simulink library "Kitchen_Lib"  (R2023a)
settings: Solver=VariableStepAuto  StartTime=0.0  StopTime=10.0  RelTol=1e-3  EnableMultiTasking=on
undefined symbols (not defined in the file): Kitc_BusTyp_P, Kitc_BusTypSkyr_C, Kitc_ColrLedColrls_C, Kitc_ColrLedGrn_C, Kitc_ColrLedRed_C, Kitc_ColrLedYlw_C, Kitc_StDgnWtrTank_C, Kitc_StElecPlugScktOffByClmp50_P, Kitc_StsDlyBlink_C, Kitc_StsErrBlink_C, Kitc_StsFctAcvn_P, Kitc_StsInfoBlink_C, Kitc_StsKitchnOffAutoIgOff_P, Kitc_StsKitchnOffBySwt_P, Kitc_StsKitchnOffDoorLockd_P, Kitc_StsKitchnOffIgOff_P, Kitc_StsKitchnOffUv_P, Kitc_StsKitchnOnBySwt_P, Kitc_StsKitchnOnNVM_P, Kitc_StsLedOff_C, Kitc_StsLedOn_C, Kitc_StsLrgCnsAcv_P, Kitc_StTrfrAnSwtInstd_P, Kitc_StTrfrSwtInstd_P, Kitc_TiKitcRefgtrOffDly_P, Kitc_ULowrThdBat_C, Kitc_UUpprThdBat_C, Kitc_ValFalse_C, Kitc_ValPwmFreq2_C, Kitc_ValPwmFreq_C, Kitc_ValTrue_C
libraries: MAN_Library x50, E2E_Lib x3
(part 6 of 13)

== system Kitchen_Lib/Kitchen/100ms/Kitchn/Subsystem1/Subsystem19/KitchenEnable/KitchenOnBySwitch ==
  Kitc_StKitcSwtUpprPart : Inport
  "GW_ModeExbn " : Inport  Port=2
  "GW_StUvTopPrio " : Inport  Port=3
  Kitchn_On : Inport  Port=4
  Logical Operator : Logic  Inputs=4  AllPortsSameDT=off  OutDataTypeStr=boolean
  Logical Operator1 : Logic  Operator=NOT  Inputs=4  AllPortsSameDT=off  OutDataTypeStr=boolean
  Logical Operator2 : Logic  Operator=NOT  Inputs=4  AllPortsSameDT=off  OutDataTypeStr=boolean
  Logical Operator3 : Logic  Operator=NOT  Inputs=4  AllPortsSameDT=off  OutDataTypeStr=boolean
  "KitchnOnBySwt " : Outport
  tag scope: Kitc_StKitcSwtUpprPart=global
  wires:
  Kitc_StKitcSwtUpprPart/1 -> [Kitc_StKitcSwtUpprPart], Logical Operator/1
  "GW_StUvTopPrio "/1 -> Logical Operator2/1
  Logical Operator/1 -> "KitchnOnBySwt "/1
  "GW_ModeExbn "/1 -> Logical Operator1/1
  Logical Operator2/1 -> Logical Operator/3
  Logical Operator3/1 -> Logical Operator/4
  Logical Operator1/1 -> Logical Operator/2
  Kitchn_On/1 -> Logical Operator3/1

== system Kitchen_Lib/Kitchen/100ms/Kitchn/Subsystem1/Subsystem19/KitchenEnable/KitchenOnNVM ==
  "GW_StStrtNew " : Inport
  "GW_ModeExbn " : Inport  Port=2
  GW_StClmp15 : Inport  Port=3
  Kitchen_On : Inport  Port=4
  KitchnOffBySwt : Inport  Port=5
  HostsSideBotmBtn_OFF : Inport  Port=6
  Kitc_ModeKitcNv : DataStoreWrite  DataStoreName=Kitc_ModeKitcNv  IndexOptions=Index vector (dialog)  Indices=1  OutputSizes=1
  Kitc_ModeKitcNv1 : DataStoreRead  DataStoreName=Kitc_ModeKitcNv  IndexOptions=Index vector (dialog)  Indices=1  OutputSizes=1
  Logical Operator32 : Logic  Inputs=5  AllPortsSameDT=off  OutDataTypeStr=boolean
  Logical Operator33 : Logic  Operator=NOT  Inputs=4  AllPortsSameDT=off  OutDataTypeStr=boolean
  Logical Operator34 : Logic  Operator=NOT  Inputs=4  AllPortsSameDT=off  OutDataTypeStr=boolean
  Logical Operator35 : Logic  Operator=NOT  Inputs=4  AllPortsSameDT=off  OutDataTypeStr=boolean
  NVM : Subsystem
  NvM_ActiveOnlyForFirstCycle : Subsystem  AncestorBlock=MAN_Library/NvM_ActiveOnlyForFirstCycle
  RisingEdgeDetection5 : Subsystem  AncestorBlock=MAN_Library/RisingEdgeDetection
  "KitchnOnNVM  " : Outport
  wires:
  "GW_ModeExbn "/1 -> Logical Operator34/1
  Logical Operator33/1 -> Logical Operator32/2
  RisingEdgeDetection5/1(Q) -> Logical Operator32/1
  Logical Operator35/1 -> Logical Operator32/5
  "GW_StStrtNew "/1 -> NVM/3("GW_StStrtNew "), Logical Operator35/1
  Logical Operator34/1 -> Logical Operator32/3
  Logical Operator32/1 -> Kitc_ModeKitcNv/1, "KitchnOnNVM  "/1
  Kitchen_On/1 -> Logical Operator33/1, NVM/5(Kitchn_On)
  Kitc_ModeKitcNv1/1 -> NvM_ActiveOnlyForFirstCycle/1(NVM_Bool_In)
  GW_StClmp15/1 -> RisingEdgeDetection5/1(CLK), NVM/6(GW_StClmp15)
  KitchnOffBySwt/1 -> NVM/1(KitchnOffBySwt)
  HostsSideBotmBtn_OFF/1 -> NVM/2(HostsSideBotmBtn_OFF)
  NvM_ActiveOnlyForFirstCycle/1(NVM_Bool_Out) -> NVM/4(Kitc_ModeKitcNv), Logical Operator32/4

== system Kitchen_Lib/Kitchen/100ms/Kitchn/Subsystem1/Subsystem19/KitchenEnable/Subsystem ==
  StateChange : Inport
  Ground : Ground
  Logical Operator : Logic  AllPortsSameDT=off  OutDataTypeStr=boolean
  RS : Subsystem  AncestorBlock=MAN_Library/RS
  RisingEdgeDetection : Subsystem  AncestorBlock=MAN_Library/RisingEdgeDetection
  StateChangePulse : Subsystem  AncestorBlock=MAN_Library/StateChangePulse
  Terminator : Terminator
  Terminator1 : Terminator
  TimeConstant : Subsystem  AncestorBlock=MAN_Library/TimeConstant  mask{hours=0, minutes=0, seconds=0, miliseconds=0}
      mask prompts: hours "Hour"
      mask DialogControl TimeConstant Prompt: Time Constant
      mask Display:
      | timeDraw = 'Time#';
      | if( hours == 0 && minutes == 0 && seconds == 0 && miliseconds == 0)
      |     timeDraw = strcat(timeDraw,'0secs'),
      | else
      |     if( hours ~= 0)
      |         timeDraw = strcat(timeDraw,num2str(hours),'hours');
      |     end
      |     if( minutes ~= 0)
      |         timeDraw = strcat(timeDraw,num2str(minutes),'min');
      |     end
      |     if( seconds ~= 0)
      |         timeDraw = strcat(timeDraw,num2str(seconds),'sec');
      |     end
      |     if( miliseconds ~= 0)
      |         timeDraw = strcat(timeDraw,num2str(miliseconds),'ms');
      |     end
      | end
      | fprintf(timeDraw);
  TurnOnDelay : Subsystem  AncestorBlock=MAN_Library/TurnOnDelay  mask(Turn On Delay){CycleTime=Cycle Time: 10 Ms}
      mask prompts: CycleTime "Select the Cycle Time:"
      mask help:
      | This is an EDGE DELAY where the turning-on edge is delayed. The delay period is entered at input PT. Output Q is set on TRUE after turning on input IN, only after the delay period is over. Output ET counts the time - beginning with the occurrence of the positive edge - until the value set at PT has been reached. The output ET shows the expired time since turning input IN on until the input state of IN is put through to output Q.
      |
      | IN : Timer starting bit
      | PT : Preset time of timer
      | Q  : Time up flag
      | ET : Current value of timer
      mask TypeOptions CycleTime: Cycle Time: 1 Ms | Cycle Time: 10 Ms | Cycle Time: 100 Ms | Cycle Time: 1000 Ms
      mask Display:
      | disp('{\bf\fontsize{18}Turn On Delay}', 'texmode','on');
      | 
      | port_label('input', 1,'IN');
      | port_label('input', 2,'PT');
      | port_label('output',1,'Q');
      | port_label('output',2,'ET');
  Unit Delay : UnitDelay  SampleTime=-1  HasFrameUpgradeWarning=on
  Kitchn_On : Outport
  wires:
  RS/1(Q) -> TurnOnDelay/1(TurnOnDelayEnable), Kitchn_On/1
  TimeConstant/1(time) -> TurnOnDelay/2(TurnOnDelayThreshold)
  TurnOnDelay/2(TurnOnDelayExpiredTime) -> Terminator/1
  TurnOnDelay/1(TurnOnDelayFlag) -> Unit Delay/1
  Unit Delay/1 -> Logical Operator/2
  Logical Operator/1 -> RS/2(R)
  RisingEdgeDetection/1(Q) -> Logical Operator/1, RS/1(S)
  StateChange/1 -> RisingEdgeDetection/1(CLK)
  Ground/1 -> StateChangePulse/1(IN)
  StateChangePulse/1(OUT) -> Terminator1/1

== system Kitchen_Lib/Kitchen/100ms/Kitchn/Subsystem1/Subsystem19/KitchenSwtLed/HostessError ==
  HostSideButtonLock : Inport
  Kitc_WarnLrgCns : Inport  Port=2
  Kitc_BusTypSkyr : Inport  Port=3
  Logical Operator14 : Logic  AllPortsSameDT=off  OutDataTypeStr=boolean
  Logical Operator15 : Logic  Operator=NOT  Inputs=4  AllPortsSameDT=off  OutDataTypeStr=boolean
  Multiport Switch3 : MultiPortSwitch  DataPortOrder=Zero-based contiguous  Inputs=2  zeroidx=on  SaturateOnIntegerOverflow=off  InputSameDT=off
  HosstesErr : Outport
  wires:
  Kitc_BusTypSkyr/1 -> Multiport Switch3/1
  HostSideButtonLock/1 -> Multiport Switch3/3, Logical Operator14/2
  Multiport Switch3/1 -> HosstesErr/1
  Logical Operator14/1 -> Multiport Switch3/2
  Logical Operator15/1 -> Logical Operator14/1
  Kitc_WarnLrgCns/1 -> Logical Operator15/1

== system Kitchen_Lib/Kitchen/100ms/Kitchn/Subsystem1/Subsystem19/KitchenSwtLed/HostessGreenDelay ==
  LrgCns : Inport
  Kitchn_On : Inport  Port=2
  Kitc_WarnLrgCns : Inport  Port=3
  HostSideButtonLock : Inport  Port=4
  HostsCallAcv : Inport  Port=5
  Kitc_BusTypSkyr : Inport  Port=6
  Constant2 : Constant  Value=Kitc_ValFalse_C
  Data Type Conversion : DataTypeConversion  OutDataTypeStr=uint8  SaturateOnIntegerOverflow=off  RndMeth=Floor
  Logical Operator{8..11} (4 alike) : Logic  Operator=NOT  Inputs=4  AllPortsSameDT=off  OutDataTypeStr=boolean
  Logical Operator7 : Logic  Inputs=5  AllPortsSameDT=off  OutDataTypeStr=boolean
  Multiport Switch4 : MultiPortSwitch  DataPortOrder=Zero-based contiguous  Inputs=2  zeroidx=on  SaturateOnIntegerOverflow=off  InputSameDT=off
  HostessGreenDly : Outport
  wires:
  Kitc_BusTypSkyr/1 -> Multiport Switch4/1
  Multiport Switch4/1 -> HostessGreenDly/1
  HostsCallAcv/1 -> Logical Operator10/1
  Kitchn_On/1 -> Logical Operator7/3
  Logical Operator8/1 -> Logical Operator7/5
  LrgCns/1 -> Logical Operator9/1
  Logical Operator9/1 -> Logical Operator7/2
  Logical Operator10/1 -> Logical Operator7/4
  Logical Operator11/1 -> Logical Operator7/1
  Kitc_WarnLrgCns/1 -> Logical Operator11/1
  Constant2/1 -> Data Type Conversion/1
  Data Type Conversion/1 -> Multiport Switch4/3
  Logical Operator7/1 -> Multiport Switch4/2
  HostSideButtonLock/1 -> Logical Operator8/1

== system Kitchen_Lib/Kitchen/100ms/Kitchn/Subsystem1/Subsystem19/KitchenSwtLed/HostessGreenOn ==
  LrgCns : Inport
  Kitchn_On : Inport  Port=2
  Kitc_WarnLrgCns : Inport  Port=3
  HostSideButtonLock : Inport  Port=4
  HostsCallAcv : Inport  Port=5
  Kitc_BusTypSkyr : Inport  Port=6
  Logical Operator1 : Logic  Inputs=4  AllPortsSameDT=off  OutDataTypeStr=boolean
  Logical Operator{2..5,54} (5 alike) : Logic  Operator=NOT  Inputs=4  AllPortsSameDT=off  OutDataTypeStr=boolean
  Logical Operator52 : Logic  Inputs=3  AllPortsSameDT=off  OutDataTypeStr=boolean
  Multiport Switch4 : MultiPortSwitch  DataPortOrder=Zero-based contiguous  Inputs=2  zeroidx=on  SaturateOnIntegerOverflow=off  InputSameDT=off
  HostessGreenOn : Outport
  wires:
  Kitc_BusTypSkyr/1 -> Multiport Switch4/1
  Multiport Switch4/1 -> HostessGreenOn/1
  HostsCallAcv/1 -> Logical Operator54/1, Logical Operator3/1
  Kitchn_On/1 -> Logical Operator52/1
  Logical Operator52/1 -> Multiport Switch4/3
  Logical Operator54/1 -> Logical Operator52/3
  HostSideButtonLock/1 -> Logical Operator5/1, Logical Operator4/1
  Logical Operator1/1 -> Multiport Switch4/2
  LrgCns/1 -> Logical Operator1/1
  Logical Operator2/1 -> Logical Operator1/2
  Logical Operator3/1 -> Logical Operator1/3
  Kitc_WarnLrgCns/1 -> Logical Operator2/1
  Logical Operator4/1 -> Logical Operator1/4
  Logical Operator5/1 -> Logical Operator52/2

== system Kitchen_Lib/Kitchen/100ms/Kitchn/Subsystem1/Subsystem19/KitchenSwtLed/HostessRed ==
  Kitc_WarnLrgCns : Inport
  HostSideButtonLock : Inport  Port=2
  HostsCallAcv : Inport  Port=3
  Kitc_BusTypSkyr : Inport  Port=4
  Logical Operator12 : Logic  AllPortsSameDT=off  OutDataTypeStr=boolean
  Logical Operator13 : Logic  Operator=NOT  Inputs=4  AllPortsSameDT=off  OutDataTypeStr=boolean
  Logical Operator5 : Logic  AllPortsSameDT=off  OutDataTypeStr=boolean
  Logical Operator8 : Logic  Operator=NOT  Inputs=4  AllPortsSameDT=off  OutDataTypeStr=boolean
  Multiport Switch4 : MultiPortSwitch  DataPortOrder=Zero-based contiguous  Inputs=2  zeroidx=on  SaturateOnIntegerOverflow=off  InputSameDT=off
  HostessRed : Outport
  wires:
  Kitc_BusTypSkyr/1 -> Multiport Switch4/1
  Multiport Switch4/1 -> HostessRed/1
  Logical Operator5/1 -> Multiport Switch4/3, Logical Operator12/2
  HostsCallAcv/1 -> Logical Operator5/1
  Logical Operator8/1 -> Logical Operator5/2
  Logical Operator12/1 -> Multiport Switch4/2
  Logical Operator13/1 -> Logical Operator12/1
  Kitc_WarnLrgCns/1 -> Logical Operator13/1
  HostSideButtonLock/1 -> Logical Operator8/1

== system Kitchen_Lib/Kitchen/100ms/Kitchn/Subsystem1/Subsystem19/KitchenSwtLed/KitchenError ==
  note: TFoE
  "GW_ModeExbn " : Inport
  "GW_StUvTopPrio " : Inport  Port=2
  In3 : Inport  Port=3
  Kitc_StKitcSwtUpprPart : Inport  Port=4
  Kitc_WarnLrgCns : Inport  Port=5
  Kitc_BusTypSkyr : Inport  Port=6
  Logical Operator21 : Logic  Operator=NOT  Inputs=4  AllPortsSameDT=off  OutDataTypeStr=boolean
  Logical Operator22 : Logic  AllPortsSameDT=off  OutDataTypeStr=boolean
  Logical Operator23 : Logic  Operator=NOT  Inputs=4  AllPortsSameDT=off  OutDataTypeStr=boolean
  Logical Operator4 : Logic  Inputs=3  AllPortsSameDT=off  OutDataTypeStr=boolean
  Multiport Switch6 : MultiPortSwitch  DataPortOrder=Zero-based contiguous  Inputs=2  zeroidx=on  SaturateOnIntegerOverflow=off  InputSameDT=off
  RisingEdgeDetection : Subsystem  AncestorBlock=MAN_Library/RisingEdgeDetection
  Terminator3 : Terminator
  TurnOffDelay : Subsystem  AncestorBlock=MAN_Library/TurnOffDelay  mask(Turn Off Delay){CycleTime=Cycle Time: 10 Ms}
      mask prompts: CycleTime "Select the Cycle Time:"
      mask help:
      | This is an EDGE DELAY where the turning-off edge is delayed. The delay period is entered at input PT. The output Q is reset after turning off input IN, only after the delay period is over. Output ET counts the time - beginning with the occurrence of the negative edge - until the value set at PT has been reached. The output ET shows the expired time since turning input IN off until the input state of IN is put through to output Q.
      |
      | IN : Timer starting bit
      | PT : Preset time of timer
      | Q  : Time pulse flag
      | ET : Current value of timer
      mask TypeOptions CycleTime: Cycle Time: 1 Ms | Cycle Time: 10 Ms | Cycle Time: 100 Ms | Cycle Time: 1000 Ms
      mask Display:
      | disp('{\bf\fontsize{18}Turn Off Delay}', 'texmode','on');
      | 
      | port_label('input', 1,'IN');
      | port_label('input', 2,'PT');
      | port_label('output',1,'Q');
      | port_label('output',2,'ET');
  KitchenErr : Outport
  wires:
  In3/1 -> TurnOffDelay/2(TurnOffDelayThreshold)
  TurnOffDelay/1(TurnOffDelayFlag) -> Logical Operator22/2, Multiport Switch6/3
  Kitc_StKitcSwtUpprPart/1 -> RisingEdgeDetection/1(CLK)
  "GW_StUvTopPrio "/1 -> Logical Operator4/2
  "GW_ModeExbn "/1 -> Logical Operator21/1
  Logical Operator4/1 -> TurnOffDelay/1(TurnOffDelayEnable)
  RisingEdgeDetection/1(Q) -> Logical Operator4/3
  Logical Operator21/1 -> Logical Operator4/1
  Multiport Switch6/1 -> KitchenErr/1
  Logical Operator23/1 -> Logical Operator22/1
  Logical Operator22/1 -> Multiport Switch6/2
  Kitc_WarnLrgCns/1 -> Logical Operator23/1
  Kitc_BusTypSkyr/1 -> Multiport Switch6/1
  TurnOffDelay/2(TurnOffDelayExpiredTime) -> Terminator3/1

== system Kitchen_Lib/Kitchen/100ms/Kitchn/Subsystem1/Subsystem19/KitchenSwtLed/KitchenGreenLed ==
  LrgCns : Inport
  Kitchn_On : Inport  Port=2
  Kitc_WarnLrgCns : Inport  Port=3
  Kitc_BusTypSkyr : Inport  Port=4
  Logical Operator16 : Logic  AllPortsSameDT=off  OutDataTypeStr=boolean
  Logical Operator17 : Logic  Operator=NOT  Inputs=4  AllPortsSameDT=off  OutDataTypeStr=boolean
  Multiport Switch4 : MultiPortSwitch  DataPortOrder=Zero-based contiguous  Inputs=2  zeroidx=on  SaturateOnIntegerOverflow=off  InputSameDT=off
  KitchenGreenOn : Outport
  wires:
  Kitchn_On/1 -> Multiport Switch4/3
  LrgCns/1 -> Logical Operator16/1
  Kitc_BusTypSkyr/1 -> Multiport Switch4/1
  Logical Operator16/1 -> Multiport Switch4/2
  Logical Operator17/1 -> Logical Operator16/2
  Kitc_WarnLrgCns/1 -> Logical Operator17/1
  Multiport Switch4/1 -> KitchenGreenOn/1

== system Kitchen_Lib/Kitchen/100ms/Kitchn/Subsystem1/Subsystem19/KitchenSwtLed/KitchenGreenLedDelay ==
  LrgCns : Inport
  Kitchn_On : Inport  Port=2
  Kitc_WarnLrgCns : Inport  Port=3
  Kitc_BusTypSkyr : Inport  Port=4
  Constant7 : Constant  Value=Kitc_ValFalse_C
  Data Type Conversion1 : DataTypeConversion  OutDataTypeStr=uint8  SaturateOnIntegerOverflow=off  RndMeth=Floor
  Logical Operator18 : Logic  Inputs=3  AllPortsSameDT=off  OutDataTypeStr=boolean
  Logical Operator19 : Logic  Operator=NOT  Inputs=4  AllPortsSameDT=off  OutDataTypeStr=boolean
  Logical Operator20 : Logic  Operator=NOT  Inputs=4  AllPortsSameDT=off  OutDataTypeStr=boolean
  Multiport Switch4 : MultiPortSwitch  DataPortOrder=Zero-based contiguous  Inputs=2  zeroidx=on  SaturateOnIntegerOverflow=off  InputSameDT=off
  KitchenGreenDly : Outport
  wires:
  Kitc_BusTypSkyr/1 -> Multiport Switch4/1
  Logical Operator18/1 -> Multiport Switch4/2
  Multiport Switch4/1 -> KitchenGreenDly/1
  Kitchn_On/1 -> Logical Operator18/1
  LrgCns/1 -> Logical Operator19/1
  Logical Operator19/1 -> Logical Operator18/3
  Logical Operator20/1 -> Logical Operator18/2
  Kitc_WarnLrgCns/1 -> Logical Operator20/1
  Constant7/1 -> Data Type Conversion1/1
  Data Type Conversion1/1 -> Multiport Switch4/3

== system Kitchen_Lib/Kitchen/100ms/Kitchn/Subsystem1/Subsystem19/KitchenSwtLed/KitchenYellowLed ==
  Kitc_WarnLrgCns : Inport
  Kitc_BusTypSkyr : Inport  Port=2
  Constant11 : Constant  Value=Kitc_ValFalse_C
  Data Type Conversion2 : DataTypeConversion  OutDataTypeStr=uint8  SaturateOnIntegerOverflow=off  RndMeth=Floor
  Multiport Switch7 : MultiPortSwitch  DataPortOrder=Zero-based contiguous  Inputs=2  zeroidx=on  SaturateOnIntegerOverflow=off  InputSameDT=off
  KitchenYellow : Outport
  wires:
  Kitc_BusTypSkyr/1 -> Multiport Switch7/1
  Data Type Conversion2/1 -> Multiport Switch7/3
  Multiport Switch7/1 -> KitchenYellow/1
  Kitc_WarnLrgCns/1 -> Multiport Switch7/2
  Constant11/1 -> Data Type Conversion2/1

== system Kitchen_Lib/Kitchen/100ms/Kitchn/Subsystem1/Subsystem19/KitchenSwtLed/LEDSignal_Subsytem ==
  note: Output Led SignalValue
      | Led Signal Blink Info
      | Led Signal Color Info
      |
      | 0
      | Off
      |
      | 1
      | 200/800
      |
      | green
      |
      | 2
      | 250/250
      |
      | green
      |
      | 3
      | 800/200
      |
      | green
      |
      | 4
      | 100%
      |
      | green
      |
      | 5
      | 200/800
      | yellow
      |
      | 6
      | 250/250
      | yellow
      |
      | 7
      | 800/200
      |
      | yellow
      |
      | 8
      | 100%
      |
      | yellow
      |
      | 9
      | 200/800
      | red
      |
      | 10
      | 250/250
      | red
      |
      | 11
      | 800/200
      |
      | red
      |
      | 12
      | 100%
      |
      | red
      |
      | 14
      | Error
      |
      | 15
      | NA
  note: Off
  note: Blink Info
      | Value
      |
      | Led off
      | 0
      |
      | Led on
      | 1
      |
      | Led 500ms on 500ms off
      | 2
      |
      | Led 250ms on 250ms off
      | 3
      |
      | Led200ms on 800ms off
      | 4
      |
      | Led 800ms on 200ms off
      | 5
  note: Led Info
      | Value
      |
      | Yellow
      | 2
      |
      | Green
      | 3
      |
      | Red
      | 1
  note: 800/200
  note: 500/500
  note: 200/800
  note: 250/250
  note: 100
  note: 800/200
  note: 500/500
  note: 200/800
  note: 250/250
  note: 100
  note: 800/200
  note: 500/500
  note: 200/800
  note: 250/250
  note: 100
  note: Off
  note: Off
  Color : Inport
  Status : Inport  Port=2
  Error : Inport  Port=3
  NA : Inport  Port=4
  Constant{1..5,56,61,66} (8 alike) : Constant  Value=uint8(0)
  Constant55 : Constant  Value=uint8(4)
  Constant57 : Constant  Value=uint8(2)
  Constant58 : Constant  Value=uint8(1)
  Constant59 : Constant  Value=uint8(3)
  Constant60 : Constant  Value=uint8(8)
  Constant62 : Constant  Value=uint8(6)
  Constant63 : Constant  Value=uint8(5)
  Constant64 : Constant  Value=uint8(7)
  Constant65 : Constant  Value=uint8(12)
  Constant67 : Constant  Value=uint8(10)
  Constant68 : Constant  Value=uint8(9)
  Constant69 : Constant  Value=uint8(11)
  Constant70 : Constant  Value=uint8(14)
  Constant71 : Constant  Value=uint8(16)
  Ground : Ground
  Ground1 : Ground
  Ground2 : Ground
  Multiport Switch17 : MultiPortSwitch  DataPortOrder=Zero-based contiguous  Inputs=6  DataPortForDefault=Additional data port  zeroidx=on  SaturateOnIntegerOverflow=off  InputSameDT=off
  Multiport Switch23 : MultiPortSwitch  DataPortOrder=Zero-based contiguous  Inputs=4  DataPortForDefault=Additional data port  DiagnosticForDefault=None  zeroidx=on  SaturateOnIntegerOverflow=off  InputSameDT=off
  Multiport Switch24 : MultiPortSwitch  DataPortOrder=Zero-based contiguous  Inputs=6  DataPortForDefault=Additional data port  zeroidx=on  SaturateOnIntegerOverflow=off  InputSameDT=off
  Multiport Switch25 : MultiPortSwitch  DataPortOrder=Zero-based contiguous  Inputs=6  DataPortForDefault=Additional data port  zeroidx=on  SaturateOnIntegerOverflow=off  InputSameDT=off
  Multiport Switch26 : MultiPortSwitch  DataPortOrder=Zero-based contiguous  Inputs=2  zeroidx=on  SaturateOnIntegerOverflow=off  InputSameDT=off
  Multiport Switch27 : MultiPortSwitch  DataPortOrder=Zero-based contiguous  Inputs=2  zeroidx=on  SaturateOnIntegerOverflow=off  InputSameDT=off
  Led : Outport
  wires:
  Status/1 -> Multiport Switch25/1, Multiport Switch24/1, Multiport Switch17/1
  Multiport Switch17/1 -> Multiport Switch23/5
  Multiport Switch24/1 -> Multiport Switch23/4
  Multiport Switch25/1 -> Multiport Switch23/3
  Constant1/1 -> Multiport Switch23/6
  Constant5/1 -> Multiport Switch23/2
  Constant57/1 -> Multiport Switch17/5
  Constant64/1 -> Multiport Switch24/7
  Ground1/1 -> Multiport Switch24/4
  Constant60/1 -> Multiport Switch24/3
  Constant62/1 -> Multiport Switch24/5
  Constant63/1 -> Multiport Switch24/6
  Constant61/1 -> Multiport Switch24/2
  Multiport Switch26/1 -> Multiport Switch27/2
  Multiport Switch23/1 -> Multiport Switch26/2
  Error/1 -> Multiport Switch26/1
  Constant69/1 -> Multiport Switch25/7
  Constant67/1 -> Multiport Switch25/5
  Ground2/1 -> Multiport Switch25/4
  Constant66/1 -> Multiport Switch25/2
  Constant68/1 -> Multiport Switch25/6
  Constant65/1 -> Multiport Switch25/3
  Constant70/1 -> Multiport Switch26/3
  Constant71/1 -> Multiport Switch27/3
  Color/1 -> Multiport Switch23/1
  Constant58/1 -> Multiport Switch17/6
  Constant55/1 -> Multiport Switch17/3
  NA/1 -> Multiport Switch27/1
  Constant56/1 -> Multiport Switch17/2
  Ground/1 -> Multiport Switch17/4
  Constant59/1 -> Multiport Switch17/7
  Multiport Switch27/1 -> Led/1
  Constant2/1 -> Multiport Switch24/8
  Constant3/1 -> Multiport Switch17/8
  Constant4/1 -> Multiport Switch25/8

== system Kitchen_Lib/Kitchen/100ms/Kitchn/Subsystem1/Subsystem19/KitchenSwtLed/LEDSignal_Subsytem1 ==
  note: Output Led SignalValue
      | Led Signal Blink Info
      | Led Signal Color Info
      |
      | 0
      | Off
      |
      | 1
      | 200/800
      |
      | green
      |
      | 2
      | 250/250
      |
      | green
      |
      | 3
      | 800/200
      |
      | green
      |
      | 4
      | 100%
      |
      | green
      |
      | 5
      | 200/800
      | yellow
      |
      | 6
      | 250/250
      | yellow
      |
      | 7
      | 800/200
      |
      | yellow
      |
      | 8
      | 100%
      |
      | yellow
      |
      | 9
      | 200/800
      | red
      |
      | 10
      | 250/250
      | red
      |
      | 11
      | 800/200
      |
      | red
      |
      | 12
      | 100%
      |
      | red
      |
      | 14
      | Error
      |
      | 15
      | NA
  note: Off
  note: Blink Info
      | Value
      |
      | Led off
      | 0
      |
      | Led on
      | 1
      |
      | Led 500ms on 500ms off
      | 2
      |
      | Led 250ms on 250ms off
      | 3
      |
      | Led200ms on 800ms off
      | 4
      |
      | Led 800ms on 200ms off
      | 5
  note: Led Info
      | Value
      |
      | Yellow
      | 2
      |
      | Green
      | 3
      |
      | Red
      | 1
  note: 800/200
  note: 500/500
  note: 200/800
  note: 250/250
  note: 100
  note: 800/200
  note: 500/500
  note: 200/800
  note: 250/250
  note: 100
  note: 800/200
  note: 500/500
  note: 200/800
  note: 250/250
  note: 100
  note: Off
  note: Off
  Color : Inport
  Status : Inport  Port=2
  Error : Inport  Port=3
  NA : Inport  Port=4
  Constant{1..5,56,61,66} (8 alike) : Constant  Value=uint8(0)
  Constant55 : Constant  Value=uint8(4)
  Constant57 : Constant  Value=uint8(2)
  Constant58 : Constant  Value=uint8(1)
  Constant59 : Constant  Value=uint8(3)
  Constant60 : Constant  Value=uint8(8)
  Constant62 : Constant  Value=uint8(6)
  Constant63 : Constant  Value=uint8(5)
  Constant64 : Constant  Value=uint8(7)
  Constant65 : Constant  Value=uint8(12)
  Constant67 : Constant  Value=uint8(10)
  Constant68 : Constant  Value=uint8(9)
  Constant69 : Constant  Value=uint8(11)
  Constant70 : Constant  Value=uint8(14)
  Constant71 : Constant  Value=uint8(16)
  Ground : Ground
  Ground1 : Ground
  Ground2 : Ground
  Multiport Switch17 : MultiPortSwitch  DataPortOrder=Zero-based contiguous  Inputs=6  DataPortForDefault=Additional data port  zeroidx=on  SaturateOnIntegerOverflow=off  InputSameDT=off
  Multiport Switch23 : MultiPortSwitch  DataPortOrder=Zero-based contiguous  Inputs=4  DataPortForDefault=Additional data port  DiagnosticForDefault=None  zeroidx=on  SaturateOnIntegerOverflow=off  InputSameDT=off
  Multiport Switch24 : MultiPortSwitch  DataPortOrder=Zero-based contiguous  Inputs=6  DataPortForDefault=Additional data port  zeroidx=on  SaturateOnIntegerOverflow=off  InputSameDT=off
  Multiport Switch25 : MultiPortSwitch  DataPortOrder=Zero-based contiguous  Inputs=6  DataPortForDefault=Additional data port  zeroidx=on  SaturateOnIntegerOverflow=off  InputSameDT=off
  Multiport Switch26 : MultiPortSwitch  DataPortOrder=Zero-based contiguous  Inputs=2  zeroidx=on  SaturateOnIntegerOverflow=off  InputSameDT=off
  Multiport Switch27 : MultiPortSwitch  DataPortOrder=Zero-based contiguous  Inputs=2  zeroidx=on  SaturateOnIntegerOverflow=off  InputSameDT=off
  Led : Outport
  wires:
  Status/1 -> Multiport Switch25/1, Multiport Switch24/1, Multiport Switch17/1
  Multiport Switch17/1 -> Multiport Switch23/5
  Multiport Switch24/1 -> Multiport Switch23/4
  Multiport Switch25/1 -> Multiport Switch23/3
  Constant1/1 -> Multiport Switch23/6
  Constant5/1 -> Multiport Switch23/2
  Constant57/1 -> Multiport Switch17/5
  Constant64/1 -> Multiport Switch24/7
  Ground1/1 -> Multiport Switch24/4
  Constant60/1 -> Multiport Switch24/3
  Constant62/1 -> Multiport Switch24/5
  Constant63/1 -> Multiport Switch24/6
  Constant61/1 -> Multiport Switch24/2
  Multiport Switch26/1 -> Multiport Switch27/2
  Multiport Switch23/1 -> Multiport Switch26/2
  Error/1 -> Multiport Switch26/1
  Constant69/1 -> Multiport Switch25/7
  Constant67/1 -> Multiport Switch25/5
  Ground2/1 -> Multiport Switch25/4
  Constant66/1 -> Multiport Switch25/2
  Constant68/1 -> Multiport Switch25/6
  Constant65/1 -> Multiport Switch25/3
  Constant70/1 -> Multiport Switch26/3
  Constant71/1 -> Multiport Switch27/3
  Color/1 -> Multiport Switch23/1
  Constant58/1 -> Multiport Switch17/6
  Constant55/1 -> Multiport Switch17/3
  NA/1 -> Multiport Switch27/1
  Constant56/1 -> Multiport Switch17/2
  Ground/1 -> Multiport Switch17/4
  Constant59/1 -> Multiport Switch17/7
  Multiport Switch27/1 -> Led/1
  Constant2/1 -> Multiport Switch24/8
  Constant3/1 -> Multiport Switch17/8
  Constant4/1 -> Multiport Switch25/8

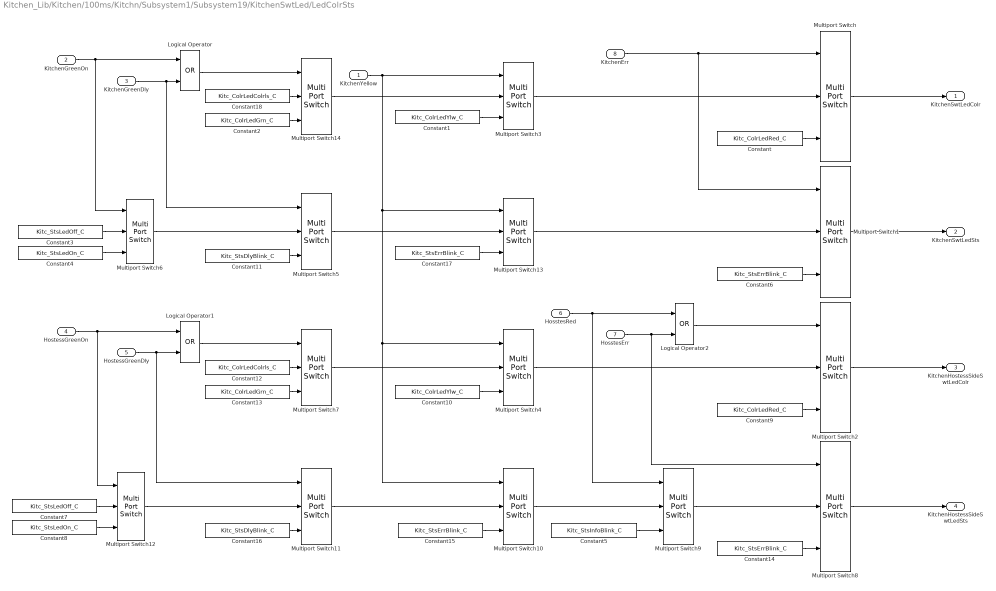
== system Kitchen_Lib/Kitchen/100ms/Kitchn/Subsystem1/Subsystem19/KitchenSwtLed/LedColrSts ==
  KitchenYellow : Inport
  KitchenGreenOn : Inport  Port=2
  KitchenGreenDly : Inport  Port=3
  HostessGreenOn : Inport  Port=4
  HostessGreenDly : Inport  Port=5
  HosstesRed : Inport  Port=6
  HosstesErr : Inport  Port=7
  KitchenErr : Inport  Port=8
  Constant : Constant  Value=Kitc_ColrLedRed_C
  Constant1 : Constant  Value=Kitc_ColrLedYlw_C
  Constant10 : Constant  Value=Kitc_ColrLedYlw_C
  Constant11 : Constant  Value=Kitc_StsDlyBlink_C
  Constant12 : Constant  Value=Kitc_ColrLedColrls_C
  Constant13 : Constant  Value=Kitc_ColrLedGrn_C
  Constant{6,14..15,17} (4 alike) : Constant  Value=Kitc_StsErrBlink_C
  Constant16 : Constant  Value=Kitc_StsDlyBlink_C
  Constant18 : Constant  Value=Kitc_ColrLedColrls_C
  Constant2 : Constant  Value=Kitc_ColrLedGrn_C
  Constant3 : Constant  Value=Kitc_StsLedOff_C
  Constant4 : Constant  Value=Kitc_StsLedOn_C
  Constant5 : Constant  Value=Kitc_StsInfoBlink_C
  Constant7 : Constant  Value=Kitc_StsLedOff_C
  Constant8 : Constant  Value=Kitc_StsLedOn_C
  Constant9 : Constant  Value=Kitc_ColrLedRed_C
  Logical Operator : Logic  Operator=OR  AllPortsSameDT=off  OutDataTypeStr=boolean
  Logical Operator1 : Logic  Operator=OR  AllPortsSameDT=off  OutDataTypeStr=boolean
  Logical Operator2 : Logic  Operator=OR  AllPortsSameDT=off  OutDataTypeStr=boolean
  Multiport Switch{,1..14} (15 alike) : MultiPortSwitch  DataPortOrder=Zero-based contiguous  Inputs=2  zeroidx=on  SaturateOnIntegerOverflow=off  InputSameDT=off
  KitchenSwtLedColr : Outport
  KitchenSwtLedSts : Outport  Port=2
  KitchenHostessSideSwtLedColr : Outport  Port=3
  KitchenHostessSideSwtLedSts : Outport  Port=4
  wires:
  Multiport Switch/1 -> KitchenSwtLedColr/1
  Multiport Switch1/1 -> KitchenSwtLedSts/1
  Multiport Switch2/1 -> KitchenHostessSideSwtLedColr/1
  Constant/1 -> Multiport Switch/3
  Multiport Switch3/1 -> Multiport Switch/2
  Constant2/1 -> Multiport Switch14/3
  Constant1/1 -> Multiport Switch3/3
  KitchenGreenOn/1 -> Logical Operator/1, Multiport Switch6/1
  Multiport Switch4/1 -> Multiport Switch2/2
  HosstesRed/1 -> Multiport Switch9/1, Logical Operator2/1
  Constant9/1 -> Multiport Switch2/3
  Constant10/1 -> Multiport Switch4/3
  KitchenGreenDly/1 -> Logical Operator/2, Multiport Switch5/1
  Logical Operator/1 -> Multiport Switch14/1
  Constant6/1 -> Multiport Switch1/3
  Multiport Switch5/1 -> Multiport Switch13/2
  Constant11/1 -> Multiport Switch5/3
  Multiport Switch6/1 -> Multiport Switch5/2
  Constant4/1 -> Multiport Switch6/3
  Constant3/1 -> Multiport Switch6/2
  KitchenYellow/1 -> Multiport Switch3/1, Multiport Switch10/1, Multiport Switch4/1, Multiport Switch13/1
  Multiport Switch7/1 -> Multiport Switch4/2
  HostessGreenOn/1 -> Logical Operator1/1, Multiport Switch12/1
  HostessGreenDly/1 -> Logical Operator1/2, Multiport Switch11/1
  Logical Operator1/1 -> Multiport Switch7/1
  Constant12/1 -> Multiport Switch7/2
  Constant13/1 -> Multiport Switch7/3
  Multiport Switch8/1 -> KitchenHostessSideSwtLedSts/1
  Multiport Switch9/1 -> Multiport Switch8/2
  Constant14/1 -> Multiport Switch8/3
  Logical Operator2/1 -> Multiport Switch2/1
  HosstesErr/1 -> Logical Operator2/2, Multiport Switch8/1
  Constant5/1 -> Multiport Switch9/3
  Multiport Switch10/1 -> Multiport Switch9/2
  Constant15/1 -> Multiport Switch10/3
  Multiport Switch11/1 -> Multiport Switch10/2
  Constant16/1 -> Multiport Switch11/3
  Multiport Switch12/1 -> Multiport Switch11/2
  Constant7/1 -> Multiport Switch12/2
  Constant8/1 -> Multiport Switch12/3
  Multiport Switch13/1 -> Multiport Switch1/2
  Multiport Switch14/1 -> Multiport Switch3/2
  KitchenErr/1 -> Multiport Switch/1, Multiport Switch1/1
  Constant17/1 -> Multiport Switch13/3
  Constant18/1 -> Multiport Switch14/2

== system Kitchen_Lib/Kitchen/100ms/Kitchn/Subsystem1/Subsystem19/KitchenSwtLed/TurnOffDelay1 ==
  TurnOffDelayEnable : Inport
  TurnOffDelayThreshold : Inport  Port=2
  Constant1 : Constant  Value=uint32(100)  OutDataTypeStr=uint32
  Constant10 : Constant  Value=uint32(CycleTime)  OutDataTypeStr=uint32
  Constant11 : Constant  Value=uint32(1)  OutDataTypeStr=uint32
  Constant12 : Constant  Value=uint32(10)  OutDataTypeStr=uint32
  Constant13 : Constant  Value=uint32(100)  OutDataTypeStr=uint32
  Constant14 : Constant  Value=uint32(1000)  OutDataTypeStr=uint32
  Multiport Switch2 : MultiPortSwitch  Inputs=4  SaturateOnIntegerOverflow=off  InputSameDT=off
  Terminator : Terminator
  TurnOffDelayOriginal : Subsystem  AncestorBlock=MAN_Library/BasicLibrary/TurnOffDelayOriginal
  TurnOffDelayFlag : Outport
  TurnOffDelayExpiredTime : Outport  Port=2
  wires:
  TurnOffDelayOriginal/2(TurnOffDelayExpiredTime) -> TurnOffDelayExpiredTime/1
  TurnOffDelayOriginal/1(TurnOffDelayFlag) -> TurnOffDelayFlag/1
  TurnOffDelayThreshold/1 -> TurnOffDelayOriginal/2(TurnOffDelayThreshold)
  TurnOffDelayEnable/1 -> TurnOffDelayOriginal/1(TurnOffDelayEnable)
  Constant11/1 -> Multiport Switch2/2
  Constant12/1 -> Multiport Switch2/3
  Constant14/1 -> Multiport Switch2/5
  Constant13/1 -> Multiport Switch2/4
  Constant10/1 -> Multiport Switch2/1
  Multiport Switch2/1 -> Terminator/1
  Constant1/1 -> TurnOffDelayOriginal/3(CycleTime)

== system Kitchen_Lib/Kitchen/100ms/Kitchn/Subsystem1/Subsystem19/Refgtr/TurnOffDelay ==
  TurnOffDelayEnable : Inport
  TurnOffDelayThreshold : Inport  Port=2
  Constant1 : Constant  Value=uint32(100)  OutDataTypeStr=uint32
  Constant10 : Constant  Value=uint32(CycleTime)  OutDataTypeStr=uint32
  Constant11 : Constant  Value=uint32(1)  OutDataTypeStr=uint32
  Constant12 : Constant  Value=uint32(10)  OutDataTypeStr=uint32
  Constant13 : Constant  Value=uint32(100)  OutDataTypeStr=uint32
  Constant14 : Constant  Value=uint32(1000)  OutDataTypeStr=uint32
  Multiport Switch2 : MultiPortSwitch  Inputs=4  SaturateOnIntegerOverflow=off  InputSameDT=off
  Terminator : Terminator
  TurnOffDelayOriginal : Subsystem  AncestorBlock=MAN_Library/BasicLibrary/TurnOffDelayOriginal
  TurnOffDelayFlag : Outport
  TurnOffDelayExpiredTime : Outport  Port=2
  wires:
  TurnOffDelayOriginal/2(TurnOffDelayExpiredTime) -> TurnOffDelayExpiredTime/1
  TurnOffDelayOriginal/1(TurnOffDelayFlag) -> TurnOffDelayFlag/1
  TurnOffDelayThreshold/1 -> TurnOffDelayOriginal/2(TurnOffDelayThreshold)
  TurnOffDelayEnable/1 -> TurnOffDelayOriginal/1(TurnOffDelayEnable)
  Constant11/1 -> Multiport Switch2/2
  Constant12/1 -> Multiport Switch2/3
  Constant14/1 -> Multiport Switch2/5
  Constant13/1 -> Multiport Switch2/4
  Constant10/1 -> Multiport Switch2/1
  Multiport Switch2/1 -> Terminator/1
  Constant1/1 -> TurnOffDelayOriginal/3(CycleTime)

== system Kitchen_Lib/Kitchen/100ms/Kitchn/Subsystem1/Subsystem19/TimePulse/TimePulseOriginal ==
  TimePulseEnable : Inport
  TimePulseDuration : Inport  Port=2
  CycleTime : Inport  Port=3
  Data Type Conversion1 : DataTypeConversion  OutDataTypeStr=uint32  SaturateOnIntegerOverflow=off  RndMeth=Floor
  Data Type Conversion2 : DataTypeConversion  OutDataTypeStr=boolean  SaturateOnIntegerOverflow=off  RndMeth=Floor
  Delay1 : Delay  DelayLength=1  InitialCondition=0  ExternalReset=Rising
      settings: InputPortMap=u0,r5
  Logical Operator1 : Logic  Operator=NOT  AllPortsSameDT=off  OutDataTypeStr=boolean
  Logical Operator2 : Logic  AllPortsSameDT=off  OutDataTypeStr=boolean
  RisingEdgeDetection : Subsystem  AncestorBlock=MAN_Library/RisingEdgeDetection
  RisingEdgeDetection1 : Subsystem  AncestorBlock=MAN_Library/RisingEdgeDetection
  SR : Subsystem  AncestorBlock=MAN_Library/SR
  TimerCountingUpOriginal : Subsystem  AncestorBlock=MAN_Library/BasicLibrary/TimerCountingUpOriginal
  TimePulseFlag : Outport
  TimePulseExpiredTime : Outport  Port=2
  wires:
  CycleTime/1 -> TimerCountingUpOriginal/4(CycleTime)
  Delay1/1 -> SR/2(R)
  [TimePulseReset] -> TimerCountingUpOriginal/2(TimerReset)
  [TimePulseReset] -> Delay1/2
  RisingEdgeDetection/1(Q) -> SR/1(S), [TimePulseReset]
  Data Type Conversion1/1 -> TimerCountingUpOriginal/3(TimerThreshold)
  Data Type Conversion2/1 -> RisingEdgeDetection/1(CLK)
  Logical Operator1/1 -> Logical Operator2/2
  Logical Operator2/1 -> TimePulseFlag/1
  RisingEdgeDetection1/1(Q) -> Delay1/1
  TimerCountingUpOriginal/1(TimerFlag) -> RisingEdgeDetection1/1(CLK), Logical Operator1/1
  SR/1(Q) -> Logical Operator2/1, TimerCountingUpOriginal/1(TimerEnable)
  TimePulseEnable/1 -> Data Type Conversion2/1
  TimePulseDuration/1 -> Data Type Conversion1/1
  TimerCountingUpOriginal/2(TimerCurrentValue) -> TimePulseExpiredTime/1

== system Kitchen_Lib/Kitchen/100ms/Kitchn/Subsystem1/Subsystem19/Trfr/001_AutomaticControlKitchenRelease ==
  Kitc_StsKitcAcv : Inport
  ABat_StAddlBatInstd : Inport  Port=2
  GW_StEngRung : Inport  Port=3
  "GW_StUvNormPrio " : Inport  Port=4
  GW_StClmp15 : Inport  Port=5
  Logical Operator : Logic  Operator=NOT  AllPortsSameDT=off  OutDataTypeStr=boolean
  Logical Operator3 : Logic  Inputs=4  AllPortsSameDT=off  OutDataTypeStr=boolean
  Logical Operator4 : Logic  Operator=OR  AllPortsSameDT=off  OutDataTypeStr=boolean
  Kitchen : Outport
  wires:
  Kitc_StsKitcAcv/1 -> Logical Operator3/1
  Logical Operator/1 -> Logical Operator3/4
  Logical Operator3/1 -> Kitchen/1
  GW_StClmp15/1 -> Logical Operator3/3
  Logical Operator4/1 -> Logical Operator3/2
  ABat_StAddlBatInstd/1 -> Logical Operator4/1
  GW_StEngRung/1 -> Logical Operator4/2
  "GW_StUvNormPrio "/1 -> Logical Operator/1

== system Kitchen_Lib/Kitchen/100ms/Kitchn/Subsystem1/Subsystem19/Trfr/002_FlipFlop ==
  GW_StClmp15 : Inport
  "GW_StUvNormPrio " : Inport  Port=2
  GW_StEngRung : Inport  Port=3
  ABat_StAddlBatInstd : Inport  Port=4
  TrfrSwt : Inport  Port=5
  Kitc_StTrfrSwtUpprPart : Inport  Port=6
  Kitc_StTrfrSwtTopBtn : Inport  Port=7
  Kitc_StTrfrSwtLowrPart : Inport  Port=8
  Kitc_StTrfrBotmBtm : Inport  Port=9
  "GW_StStrtNew " : Inport  Port=10
  Kitc_StTrfrWoutNewStrt : Inport  Port=11
  KSW-Nvm : Subsystem
  Kitc_StsTurnOnByBtnNv : DataStoreRead  DataStoreName=Kitc_StsTurnOnByBtnNv  IndexOptions=Index vector (dialog)  Indices=1  OutputSizes=1
  Logical Operator5 : Logic  Operator=OR  Inputs=4  AllPortsSameDT=off  OutDataTypeStr=boolean
  NvM_ActiveOnlyForFirstCycle : Subsystem  AncestorBlock=MAN_Library/NvM_ActiveOnlyForFirstCycle
  StateChangePulse : Subsystem  AncestorBlock=MAN_Library/StateChangePulse
  TurnOffByButton : Subsystem
  TurnOffConditions : Subsystem
  TurnOnByButton : Subsystem
  TurnOnNvm : Subsystem
  Unit Delay : UnitDelay  SampleTime=-1  HasFrameUpgradeWarning=on
  Fnc_On : Outport
  wires:
  StateChangePulse/1(OUT) -> Unit Delay/1, Fnc_On/1
  Logical Operator5/1 -> StateChangePulse/1(IN)
  Unit Delay/1 -> [Fnc_ON]
  "GW_StStrtNew "/1 -> KSW-Nvm/3("GW_StStrtNew ")
  [TurnOff] -> KSW-Nvm/2(TurnOff)
  Kitc_StTrfrWoutNewStrt/1 -> KSW-Nvm/4(Kitc_StTrfrWoutNewStrt)
  [TurnOn] -> KSW-Nvm/1(TurnOn)
  ABat_StAddlBatInstd/1 -> [ABat_StAddlBatInstd]
  GW_StEngRung/1 -> [GW_StEngRung]
  GW_StClmp15/1 -> [GW_StClmp15]
  "GW_StUvNormPrio "/1 -> [GW_StUvNormPrio]
  Kitc_StsTurnOnByBtnNv/1 -> NvM_ActiveOnlyForFirstCycle/1(NVM_Bool_In)
  TurnOnByButton/1(TurnOn) -> Logical Operator5/1, [TurnOn]
  Kitc_StTrfrSwtUpprPart/1 -> TurnOnByButton/1(Kitc_StTrfrSwtUpprPart)
  Kitc_StTrfrSwtTopBtn/1 -> TurnOnByButton/2(Kitc_StTrfrSwtTopBtn)
  TurnOffByButton/1(TurnOff) -> [TurnOff], Logical Operator5/2
  Kitc_StTrfrSwtLowrPart/1 -> TurnOffByButton/1(Kitc_StTrfrSwtLowrPart)
  Kitc_StTrfrBotmBtm/1 -> TurnOffByButton/2(Kitc_StTrfrBotmBtm)
  TurnOffConditions/1(CdnOff) -> Logical Operator5/3
  TrfrSwt/1 -> TurnOnNvm/1(TrfrSwt)
  TurnOnNvm/1(TurnOnNvm) -> Logical Operator5/4
  [Fnc_ON] -> TurnOnByButton/7(Fnc_ON)
  [Fnc_ON] -> TurnOffByButton/3(Fnc_ON)
  [GW_StUvNormPrio] -> TurnOnByButton/6("GW_StUvNormPrio ")
  [GW_StClmp15] -> TurnOnByButton/5(GW_StClmp15)
  [ABat_StAddlBatInstd] -> TurnOnByButton/4(ABat_StAddlBatInstd)
  [GW_StEngRung] -> TurnOnByButton/3(GW_StEngRung)
  [GW_StEngRung] -> TurnOffConditions/1(GW_StEngRung)
  [ABat_StAddlBatInstd] -> TurnOffConditions/2(ABat_StAddlBatInstd)
  [GW_StClmp15] -> TurnOffConditions/3(GW_StClmp15)
  [GW_StUvNormPrio] -> TurnOffConditions/4("GW_StUvNormPrio ")
  [Fnc_ON] -> TurnOffConditions/5(Fnc_ON)
  [GW_StEngRung] -> TurnOnNvm/3(GW_StEngRung)
  [ABat_StAddlBatInstd] -> TurnOnNvm/4(ABat_StAddlBatInstd)
  [GW_StClmp15] -> TurnOnNvm/5(GW_StClmp15)
  [GW_StUvNormPrio] -> TurnOnNvm/7(GW_StUvNormPrio)
  [Fnc_ON] -> TurnOnNvm/6(Fnc_ON)
  NvM_ActiveOnlyForFirstCycle/1(NVM_Bool_Out) -> TurnOnNvm/2(Kitc_StsTurnOnByBtnNv)

== system Kitchen_Lib/Kitchen/100ms/Kitchn/Subsystem1/Subsystem19/Trfr/Constant1                                                                  ==
  Constant11 : Constant  Value=uint32(hours)  OutDataTypeStr=uint32
  Constant12 : Constant  Value=uint32(minutes)  OutDataTypeStr=uint32
  Constant13 : Constant  Value=uint32(miliseconds)  OutDataTypeStr=uint32
  Constant14 : Constant  Value=uint32(60)  OutDataTypeStr=uint32
  Constant15 : Constant  Value=uint32(1000)  OutDataTypeStr=uint32
  Constant16 : Constant  Value=uint32(seconds)  OutDataTypeStr=uint32
  Constant17 : Constant  Value=uint32(1000)  OutDataTypeStr=uint32
  Constant7 : Constant  Value=uint32(60)  OutDataTypeStr=uint32
  Constant8 : Constant  Value=uint32(60)  OutDataTypeStr=uint32
  Constant9 : Constant  Value=uint32(1000)  OutDataTypeStr=uint32
  Data Type Conversion{1..2,4..8,13..19} (14 alike) : DataTypeConversion  OutDataTypeStr=uint32  SaturateOnIntegerOverflow=off  RndMeth=Floor
  Product1 : Product  Inputs=4  OutDataTypeStr=uint32
  Product2 : Product  Inputs=3  OutDataTypeStr=uint32
  Product4 : Product  OutDataTypeStr=uint32
  Sum1 : Sum  Inputs=++++  AccumDataTypeStr=uint32
  time : Outport
  wires:
  Sum1/1 -> Data Type Conversion5/1  "time"
  Data Type Conversion5/1 -> time/1
  Constant7/1 -> Data Type Conversion13/1
  Data Type Conversion13/1 -> Product1/1
  Constant8/1 -> Data Type Conversion14/1
  Data Type Conversion14/1 -> Product1/2
  Constant9/1 -> Data Type Conversion15/1
  Data Type Conversion15/1 -> Product1/3
  Constant11/1 -> Data Type Conversion16/1
  Data Type Conversion16/1 -> Product1/4
  Constant12/1 -> Data Type Conversion2/1
  Constant14/1 -> Data Type Conversion17/1
  Data Type Conversion17/1 -> Product2/1
  Constant15/1 -> Data Type Conversion18/1
  Data Type Conversion18/1 -> Product2/2
  Constant17/1 -> Data Type Conversion19/1
  Data Type Conversion19/1 -> Product4/1
  Constant16/1 -> Data Type Conversion1/1
  Product1/1 -> Data Type Conversion4/1
  Product2/1 -> Data Type Conversion6/1
  Product4/1 -> Data Type Conversion7/1
  Data Type Conversion1/1 -> Product4/2
  Data Type Conversion2/1 -> Product2/3
  Constant13/1 -> Data Type Conversion8/1
  Data Type Conversion4/1 -> Sum1/1
  Data Type Conversion6/1 -> Sum1/2
  Data Type Conversion7/1 -> Sum1/3
  Data Type Conversion8/1 -> Sum1/4

== system Kitchen_Lib/Kitchen/100ms/Kitchn/Subsystem1/Subsystem19/Trfr/TurnOnDelay ==
  TurnOnDelayEnable : Inport
  TurnOnDelayThreshold : Inport  Port=2
  Constant1 : Constant  Value=uint32(100)  OutDataTypeStr=uint32
  Constant11 : Constant  Value=uint32(1)  OutDataTypeStr=uint32
  Constant12 : Constant  Value=uint32(10)  OutDataTypeStr=uint32
  Constant13 : Constant  Value=uint32(100)  OutDataTypeStr=uint32
  Constant14 : Constant  Value=uint32(1000)  OutDataTypeStr=uint32
  Constant2 : Constant  Value=uint32(CycleTime)  OutDataTypeStr=uint32
  Multiport Switch2 : MultiPortSwitch  Inputs=4  SaturateOnIntegerOverflow=off  InputSameDT=off
  Terminator : Terminator
  TurnOnDelayOriginal : Subsystem  AncestorBlock=MAN_Library/BasicLibrary/TurnOnDelayOriginal
  TurnOnDelayFlag : Outport
  TurnOnDelayExpiredTime : Outport  Port=2
  wires:
  TurnOnDelayEnable/1 -> TurnOnDelayOriginal/1(TurnOnDelayEnable)
  TurnOnDelayThreshold/1 -> TurnOnDelayOriginal/2(TurnOnDelayThreshold)
  TurnOnDelayOriginal/2(TurnOnDelayExpiredTime) -> TurnOnDelayExpiredTime/1
  TurnOnDelayOriginal/1(TurnOnDelayFlag) -> TurnOnDelayFlag/1
  Constant11/1 -> Multiport Switch2/2
  Constant12/1 -> Multiport Switch2/3
  Constant14/1 -> Multiport Switch2/5
  Constant13/1 -> Multiport Switch2/4
  Constant2/1 -> Multiport Switch2/1
  Multiport Switch2/1 -> Terminator/1
  Constant1/1 -> TurnOnDelayOriginal/3(CycleTime)

== system Kitchen_Lib/Kitchen/100ms/Kitchn/Subsystem1/Subsystem19/WaterTankEmptyDiagnostic/Constant                                          ==
  Constant11 : Constant  Value=uint32(hours)  OutDataTypeStr=uint32
  Constant12 : Constant  Value=uint32(minutes)  OutDataTypeStr=uint32
  Constant13 : Constant  Value=uint32(miliseconds)  OutDataTypeStr=uint32
  Constant14 : Constant  Value=uint32(60)  OutDataTypeStr=uint32
  Constant15 : Constant  Value=uint32(1000)  OutDataTypeStr=uint32
  Constant16 : Constant  Value=uint32(seconds)  OutDataTypeStr=uint32
  Constant17 : Constant  Value=uint32(1000)  OutDataTypeStr=uint32
  Constant7 : Constant  Value=uint32(60)  OutDataTypeStr=uint32
  Constant8 : Constant  Value=uint32(60)  OutDataTypeStr=uint32
  Constant9 : Constant  Value=uint32(1000)  OutDataTypeStr=uint32
  Data Type Conversion{1..2,4..8,13..19} (14 alike) : DataTypeConversion  OutDataTypeStr=uint32  SaturateOnIntegerOverflow=off  RndMeth=Floor
  Product1 : Product  Inputs=4  OutDataTypeStr=uint32
  Product2 : Product  Inputs=3  OutDataTypeStr=uint32
  Product4 : Product  OutDataTypeStr=uint32
  Sum1 : Sum  Inputs=++++  AccumDataTypeStr=uint32
  time : Outport
  wires:
  Sum1/1 -> Data Type Conversion5/1  "time"
  Data Type Conversion5/1 -> time/1
  Constant7/1 -> Data Type Conversion13/1
  Data Type Conversion13/1 -> Product1/1
  Constant8/1 -> Data Type Conversion14/1
  Data Type Conversion14/1 -> Product1/2
  Constant9/1 -> Data Type Conversion15/1
  Data Type Conversion15/1 -> Product1/3
  Constant11/1 -> Data Type Conversion16/1
  Data Type Conversion16/1 -> Product1/4
  Constant12/1 -> Data Type Conversion2/1
  Constant14/1 -> Data Type Conversion17/1
  Data Type Conversion17/1 -> Product2/1
  Constant15/1 -> Data Type Conversion18/1
  Data Type Conversion18/1 -> Product2/2
  Constant17/1 -> Data Type Conversion19/1
  Data Type Conversion19/1 -> Product4/1
  Constant16/1 -> Data Type Conversion1/1
  Product1/1 -> Data Type Conversion4/1
  Product2/1 -> Data Type Conversion6/1
  Product4/1 -> Data Type Conversion7/1
  Data Type Conversion1/1 -> Product4/2
  Data Type Conversion2/1 -> Product2/3
  Constant13/1 -> Data Type Conversion8/1
  Data Type Conversion4/1 -> Sum1/1
  Data Type Conversion6/1 -> Sum1/2
  Data Type Conversion7/1 -> Sum1/3
  Data Type Conversion8/1 -> Sum1/4

== system Kitchen_Lib/Kitchen/100ms/Kitchn/Subsystem1/Subsystem19/WaterTankEmptyDiagnostic/Constant1                                         ==
  Constant11 : Constant  Value=uint32(hours)  OutDataTypeStr=uint32
  Constant12 : Constant  Value=uint32(minutes)  OutDataTypeStr=uint32
  Constant13 : Constant  Value=uint32(miliseconds)  OutDataTypeStr=uint32
  Constant14 : Constant  Value=uint32(60)  OutDataTypeStr=uint32
  Constant15 : Constant  Value=uint32(1000)  OutDataTypeStr=uint32
  Constant16 : Constant  Value=uint32(seconds)  OutDataTypeStr=uint32
  Constant17 : Constant  Value=uint32(1000)  OutDataTypeStr=uint32
  Constant7 : Constant  Value=uint32(60)  OutDataTypeStr=uint32
  Constant8 : Constant  Value=uint32(60)  OutDataTypeStr=uint32
  Constant9 : Constant  Value=uint32(1000)  OutDataTypeStr=uint32
  Data Type Conversion{1..2,4..8,13..19} (14 alike) : DataTypeConversion  OutDataTypeStr=uint32  SaturateOnIntegerOverflow=off  RndMeth=Floor
  Product1 : Product  Inputs=4  OutDataTypeStr=uint32
  Product2 : Product  Inputs=3  OutDataTypeStr=uint32
  Product4 : Product  OutDataTypeStr=uint32
  Sum1 : Sum  Inputs=++++  AccumDataTypeStr=uint32
  time : Outport
  wires:
  Sum1/1 -> Data Type Conversion5/1  "time"
  Data Type Conversion5/1 -> time/1
  Constant7/1 -> Data Type Conversion13/1
  Data Type Conversion13/1 -> Product1/1
  Constant8/1 -> Data Type Conversion14/1
  Data Type Conversion14/1 -> Product1/2
  Constant9/1 -> Data Type Conversion15/1
  Data Type Conversion15/1 -> Product1/3
  Constant11/1 -> Data Type Conversion16/1
  Data Type Conversion16/1 -> Product1/4
  Constant12/1 -> Data Type Conversion2/1
  Constant14/1 -> Data Type Conversion17/1
  Data Type Conversion17/1 -> Product2/1
  Constant15/1 -> Data Type Conversion18/1
  Data Type Conversion18/1 -> Product2/2
  Constant17/1 -> Data Type Conversion19/1
  Data Type Conversion19/1 -> Product4/1
  Constant16/1 -> Data Type Conversion1/1
  Product1/1 -> Data Type Conversion4/1
  Product2/1 -> Data Type Conversion6/1
  Product4/1 -> Data Type Conversion7/1
  Data Type Conversion1/1 -> Product4/2
  Data Type Conversion2/1 -> Product2/3
  Constant13/1 -> Data Type Conversion8/1
  Data Type Conversion4/1 -> Sum1/1
  Data Type Conversion6/1 -> Sum1/2
  Data Type Conversion7/1 -> Sum1/3
  Data Type Conversion8/1 -> Sum1/4

== system Kitchen_Lib/Kitchen/100ms/Kitchn/Subsystem1/Subsystem19/WaterTankEmptyDiagnostic/Constant2                                         ==
  Constant11 : Constant  Value=uint32(hours)  OutDataTypeStr=uint32
  Constant12 : Constant  Value=uint32(minutes)  OutDataTypeStr=uint32
  Constant13 : Constant  Value=uint32(miliseconds)  OutDataTypeStr=uint32
  Constant14 : Constant  Value=uint32(60)  OutDataTypeStr=uint32
  Constant15 : Constant  Value=uint32(1000)  OutDataTypeStr=uint32
  Constant16 : Constant  Value=uint32(seconds)  OutDataTypeStr=uint32
  Constant17 : Constant  Value=uint32(1000)  OutDataTypeStr=uint32
  Constant7 : Constant  Value=uint32(60)  OutDataTypeStr=uint32
  Constant8 : Constant  Value=uint32(60)  OutDataTypeStr=uint32
  Constant9 : Constant  Value=uint32(1000)  OutDataTypeStr=uint32
  Data Type Conversion{1..2,4..8,13..19} (14 alike) : DataTypeConversion  OutDataTypeStr=uint32  SaturateOnIntegerOverflow=off  RndMeth=Floor
  Product1 : Product  Inputs=4  OutDataTypeStr=uint32
  Product2 : Product  Inputs=3  OutDataTypeStr=uint32
  Product4 : Product  OutDataTypeStr=uint32
  Sum1 : Sum  Inputs=++++  AccumDataTypeStr=uint32
  time : Outport
  wires:
  Sum1/1 -> Data Type Conversion5/1  "time"
  Data Type Conversion5/1 -> time/1
  Constant7/1 -> Data Type Conversion13/1
  Data Type Conversion13/1 -> Product1/1
  Constant8/1 -> Data Type Conversion14/1
  Data Type Conversion14/1 -> Product1/2
  Constant9/1 -> Data Type Conversion15/1
  Data Type Conversion15/1 -> Product1/3
  Constant11/1 -> Data Type Conversion16/1
  Data Type Conversion16/1 -> Product1/4
  Constant12/1 -> Data Type Conversion2/1
  Constant14/1 -> Data Type Conversion17/1
  Data Type Conversion17/1 -> Product2/1
  Constant15/1 -> Data Type Conversion18/1
  Data Type Conversion18/1 -> Product2/2
  Constant17/1 -> Data Type Conversion19/1
  Data Type Conversion19/1 -> Product4/1
  Constant16/1 -> Data Type Conversion1/1
  Product1/1 -> Data Type Conversion4/1
  Product2/1 -> Data Type Conversion6/1
  Product4/1 -> Data Type Conversion7/1
  Data Type Conversion1/1 -> Product4/2
  Data Type Conversion2/1 -> Product2/3
  Constant13/1 -> Data Type Conversion8/1
  Data Type Conversion4/1 -> Sum1/1
  Data Type Conversion6/1 -> Sum1/2
  Data Type Conversion7/1 -> Sum1/3
  Data Type Conversion8/1 -> Sum1/4

== system Kitchen_Lib/Kitchen/100ms/Kitchn/Subsystem1/Subsystem19/WaterTankEmptyDiagnostic/DIAG ==
  In1 : Inport
  In2 : Inport  Port=2
  Dem_SetEventStatus : MAN_Library/Dem_SetEventStatus  Commented=on  SLB_DEMEventID=Kitc_StDgnWtrTank_C
  Terminator : Terminator
  Terminator1 : Terminator
  wires:
  In1/1 -> Terminator/1
  In2/1 -> Terminator1/1
